simulink model "FrequencyConverter"  (R2025b)
settings: Solver=FixedStepAuto  StartTime=0.0  StopTime=100.0  FixedStep=Ts  RelTol=1e-3
values from neighbouring files (symbols this model uses):
  M_AD_nom = 3500.0    (= 3500)    [constants.m]
  M_max_factor = 2.2    [constants.m]
  poles = 2    [constants.m]
  s_max = 0.05    [constants.m]
settings Model: TunableVars=J_AD,J_ICE,M_AD_nom,P_ballast_nom,P_oil_max,P_oil_min,T_AD_max,T_amb,T_ballast_max,T_cool_max,a_const,ad_fun_acceleration,b_const,k_heat,k_loss,k_loss0,k_rad_AD,k_rad_ballast,k_radiator,omega_ICE_max_prir,omega_ICE_max_run,tau,tau_AD_base,tau_ballast,tau_cool  TunableVarsStorageClass=Auto,Auto,Auto,Auto,Auto,Auto,Auto,Auto,Auto,Auto,Auto,Auto,Auto,Auto,Auto,Auto,Auto,Auto,Auto,Auto,Auto,Auto,Auto,Auto,Auto  TunableVarsTypeQualifier=,,,,,,,,,,,,,,,,,,,,,,,,  Creator=user  LastModifiedBy=user
settings OptimizationCC: DefaultParameterBehavior=Inlined  UseDivisionForNetSlopeComputation=on  GainParamInheritBuiltInType=on  UseFloatMulNetSlope=on  StrengthReduction=on  PassReuseOutputArgsAs=Individual arguments  NoFixptDivByZeroProtection=on  EfficientFloat2IntCast=on  OptimizeBlockOrder=speed  OptimizationPriority=Speed  OptimizationCustomize=off  MultiThreadedLoops=on  AutoScheduleForLoops=on  EfficientTunableParamExpr=on
settings DebuggingCC: ParameterTunabilityLossMsg=error
settings HardwareCC: ProdBitPerLong=64.0  ProdLongLongMode=on  ProdHWDeviceType=Intel->x86-64 (Linux 64)
settings SFSimCC: MATLABDynamicMemAlloc=off  SimTargetLang=C++  SimDLTargetLibrary=mkl-dnn
settings RTWCC: SystemTargetFile=ert.tlc  GenCodeOnly=on  TemplateMakefile=ert_default_tmf  GenerateReport=on  BuildConfiguration=Faster Runs  LaunchReport=on  TargetLang=C++  Description=Embedded Coder
settings CodeAppCC: ForceParamTrailComments=on  IgnoreCustomStorageClasses=off  OperatorAnnotations=on  SimulinkDataObjDesc=on  SFDataObjDesc=on  CustomSymbolStrGlobalVar=rt$N$M  CustomSymbolStrType=$N$M  CustomSymbolStrFcn=$N$M$F  CustomSymbolStrMacro=$N$M  InsertBlockDesc=on
settings ERTTargetCC: InlinedParameterPlacement=Hierarchical  RootIOFormat=Structure reference  ERTCustomFileTemplate=example_file_process.tlc  TargetLangStandard=C++17 (ISO)  GenerateSampleERTMain=on  CodeInterfacePackaging=Reusable function  SupportContinuousTime=on

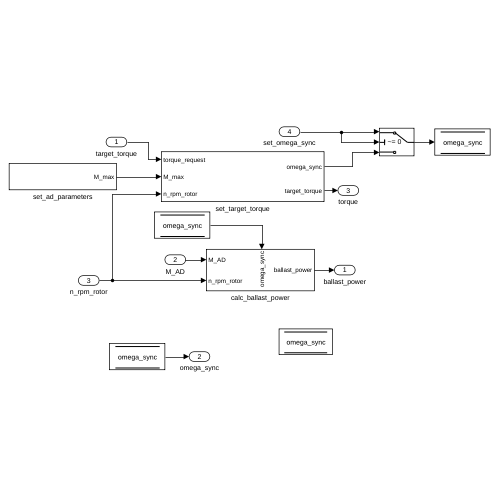
[thumbnail: Simulink's stored preview of the top-level diagram]
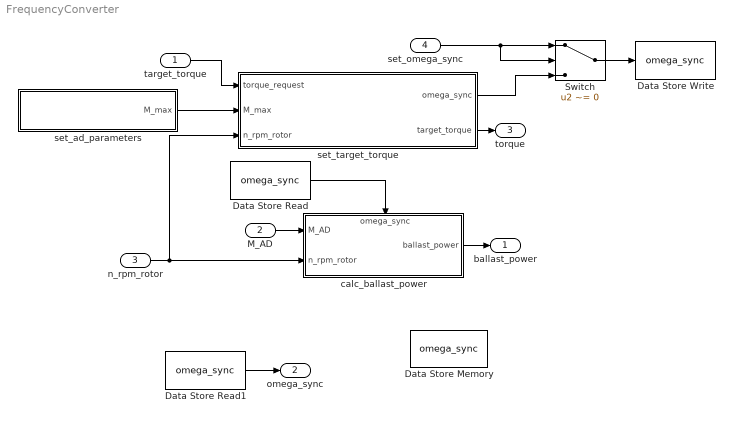
== system FrequencyConverter ==
  target_torque : Inport
  M_AD : Inport  Port=2
  n_rpm_rotor : Inport  Port=3
  set_omega_sync : Inport  Port=4
  Data Store Memory : DataStoreMemory  DataStoreName=omega_sync  WriteAfterWriteMsg=warning  ShowAdditionalParam=off
  Data Store Read : DataStoreRead  DataStoreName=omega_sync  IndexOptions=Index vector (dialog)  Indices=1  OutputSizes=1
  Data Store Read1 : DataStoreRead  DataStoreName=omega_sync  IndexOptions=Index vector (dialog)  Indices=1  OutputSizes=1
  Data Store Write : DataStoreWrite  DataStoreName=omega_sync  IndexOptions=Index vector (dialog)  Indices=1  OutputSizes=1
  Switch : Switch  Criteria=u2 ~= 0  SaturateOnIntegerOverflow=off  InputSameDT=off
  calc_ballast_power : Subsystem
      settings: PortSchema="{\"entries\":[{\"content\":{\"sides\":[{\"content\":{\"connectorIds\":[\"In1\",\"In2\"]},\"type\":\"ConnectorPlacement.EquallySpacedRectSide\",\"uuid\":\"9c23e3e7-388c-4891-afdd-4d1624b884f1\"},{\"content\":{\"connectorIds\":[\"Out1\"],\"side\":\"RIGHT\"},\"type\":\"ConnectorPlacement.EquallySpacedRectSide\",\"uuid\":\"c0260273-0b08-4e98-9658-3297e997359d\"},{\"content\":{\"connectorIds\":[\"In3\"],\"side\":\"TOP\"},\"type\":\"ConnectorPlacement.EquallySpacedRectSide\",\"uuid\":\"b122e6e2-13b5-4687-be80-e20d337b8a3a\"}]},\"type\":\"ConnectorPlacement.EquallySpacedConnector\",\"uuid\":\"625c4f0e-8d47-4f32-9019-3adc0e8607fd\"}],\"packageUris\":[\"http://schema.mathworks.com/mf0/Connector/R2020b\"],\"version\":\"1.0\"}"
  set_ad_parameters : Subsystem
  set_target_torque : Subsystem
  ballast_power : Outport
  omega_sync : Outport  Port=2
  torque : Outport  Port=3
  wires:
  M_AD/1 -> calc_ballast_power/1(M_AD)
  n_rpm_rotor/1 -> set_target_torque/3(n_rpm_rotor), calc_ballast_power/2(n_rpm_rotor)
  calc_ballast_power/1(ballast_power) -> ballast_power/1
  set_ad_parameters/1(M_max) -> set_target_torque/2(M_max)
  target_torque/1 -> set_target_torque/1(torque_request)
  Data Store Read/1 -> calc_ballast_power/3(omega_sync)
  Data Store Read1/1 -> omega_sync/1
  set_target_torque/1(omega_sync) -> Switch/3
  set_omega_sync/1 -> Switch/2, Switch/1
  Switch/1 -> Data Store Write/1
  set_target_torque/2(target_torque) -> torque/1

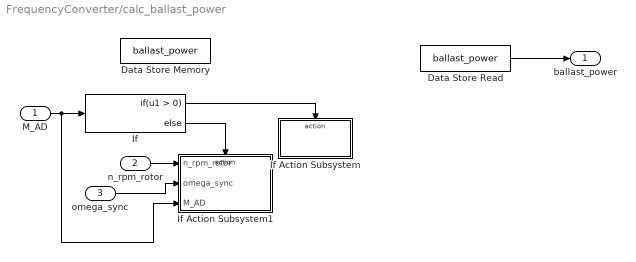
== system FrequencyConverter/calc_ballast_power ==
  M_AD : Inport
  n_rpm_rotor : Inport  Port=2
  omega_sync : Inport  Port=3
  Data Store Memory : DataStoreMemory  DataStoreName=ballast_power  WriteAfterWriteMsg=warning  ShowAdditionalParam=off
  Data Store Read : DataStoreRead  DataStoreName=ballast_power  IndexOptions=Index vector (dialog)  Indices=1  OutputSizes=1
  If : If
  If Action Subsystem : Subsystem  TreatAsAtomicUnit=on
  If Action Subsystem1 : Subsystem  TreatAsAtomicUnit=on
  ballast_power : Outport
  wires:
  Data Store Read/1 -> ballast_power/1
  M_AD/1 -> If Action Subsystem1/3(M_AD), If/1
  If/1 -> If Action Subsystem/Action
  If/2 -> If Action Subsystem1/Action
  n_rpm_rotor/1 -> If Action Subsystem1/1(n_rpm_rotor)
  omega_sync/1 -> If Action Subsystem1/2(omega_sync)

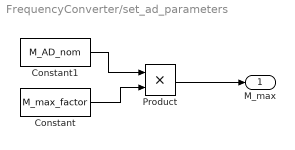
== system FrequencyConverter/set_ad_parameters ==
  Constant : Constant  Value=M_max_factor
  Constant1 : Constant  Value=M_AD_nom
  Product : Product
  M_max : Outport
  wires:
  Constant/1 -> Product/2
  Constant1/1 -> Product/1
  Product/1 -> M_max/1

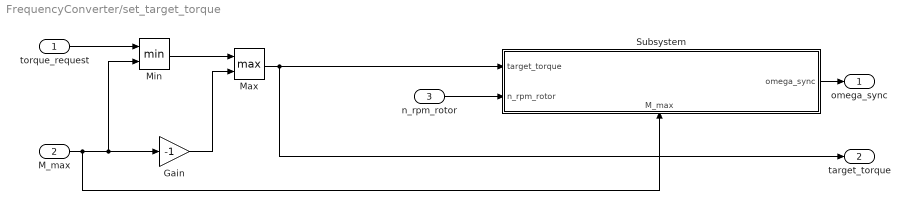
== system FrequencyConverter/set_target_torque ==
  torque_request : Inport
  M_max : Inport  Port=2
  n_rpm_rotor : Inport  Port=3
  Gain : Gain  Gain=-1
  Max : MinMax  Function=max  Inputs=2
  Min : MinMax  Inputs=2
  Subsystem : Subsystem
      settings: PortSchema="{\"entries\":[{\"content\":{\"sides\":[{\"content\":{\"connectorIds\":[\"In1\",\"In2\"]},\"type\":\"ConnectorPlacement.EquallySpacedRectSide\",\"uuid\":\"f5037b0f-1ffd-4c9a-b1c3-4b725bea221f\"},{\"content\":{\"connectorIds\":[\"Out1\"],\"side\":\"RIGHT\"},\"type\":\"ConnectorPlacement.EquallySpacedRectSide\",\"uuid\":\"2266316a-45d6-4ff2-af39-82d45dce8729\"},{\"content\":{\"side\":\"TOP\"},\"type\":\"ConnectorPlacement.EquallySpacedRectSide\",\"uuid\":\"46200062-e85d-4adb-b79b-d00d6ab0e852\"},{\"content\":{\"connectorIds\":[\"In3\"],\"side\":\"BOTTOM\"},\"type\":\"ConnectorPlacement.EquallySpacedRectSide\",\"uuid\":\"97407893-4fba-4239-999b-cdb868f8b31f\"}]},\"type\":\"ConnectorPlacement.EquallySpacedConnector\",\"uuid\":\"87dda9e4-bbd4-43d9-bcb0-f10d68c020c2\"}],\"packageUris\":[\"http://schema.mathworks.com/mf0/Connector/R2020b\"],\"version\":\"1.0\"}"
  omega_sync : Outport
  target_torque : Outport  Port=2
  wires:
  torque_request/1 -> Min/1
  M_max/1 -> Subsystem/3(M_max), Min/2, Gain/1
  Gain/1 -> Max/2
  Max/1 -> target_torque/1, Subsystem/1(target_torque)
  Min/1 -> Max/1
  Subsystem/1(omega_sync) -> omega_sync/1
  n_rpm_rotor/1 -> Subsystem/2(n_rpm_rotor)

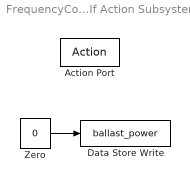
== system FrequencyConverter/calc_ballast_power/If Action Subsystem ==
  Action Port : ActionPort  ActionPortLabel=if(u1 > 0)
  Data Store Write : DataStoreWrite  DataStoreName=ballast_power  IndexOptions=Index vector (dialog)  Indices=1  OutputSizes=1
  Zero : Constant  Value=0  OutDataTypeStr=Inherit: Inherit via back propagation
  wires:
  Zero/1 -> Data Store Write/1

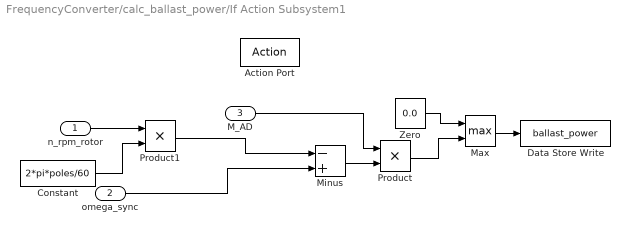
== system FrequencyConverter/calc_ballast_power/If Action Subsystem1 ==
  n_rpm_rotor : Inport
  omega_sync : Inport  Port=2
  M_AD : Inport  Port=3
  Action Port : ActionPort  ActionPortLabel=else
  Constant : Constant  Value=2*pi*poles/60
  Data Store Write : DataStoreWrite  DataStoreName=ballast_power  IndexOptions=Index vector (dialog)  Indices=1  OutputSizes=1
  Max : MinMax  Function=max  Inputs=2
  Minus : Sum  Inputs=-+
  Product : Product
  Product1 : Product
  Zero : Constant  Value=0.0  OutDataTypeStr=Inherit: Inherit via back propagation
  wires:
  Product/1 -> Max/2
  Zero/1 -> Max/1
  Minus/1 -> Product/2
  omega_sync/1 -> Minus/2
  M_AD/1 -> Product/1
  n_rpm_rotor/1 -> Product1/1
  Product1/1 -> Minus/1
  Constant/1 -> Product1/2
  Max/1 -> Data Store Write/1

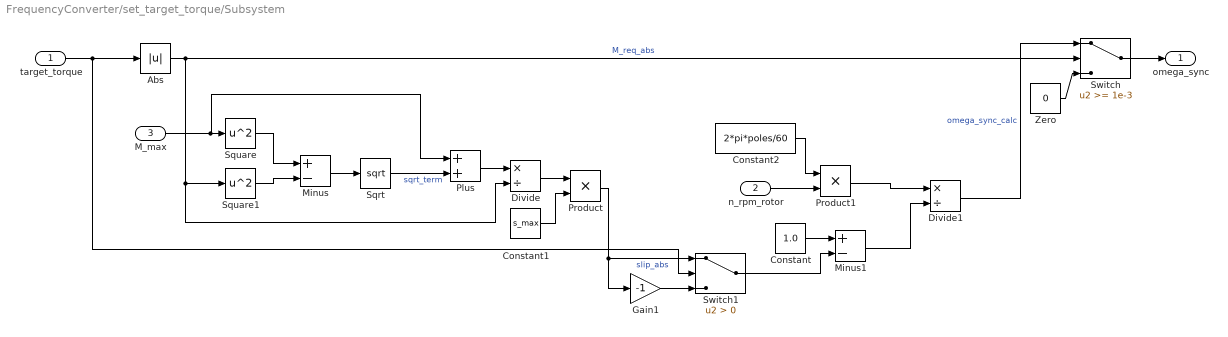
== system FrequencyConverter/set_target_torque/Subsystem ==
  target_torque : Inport
  n_rpm_rotor : Inport  Port=2
  M_max : Inport  Port=3
  Abs : Abs  SaturateOnIntegerOverflow=off
  Constant : Constant  Value=1.0
  Constant1 : Constant  Value=s_max
  Constant2 : Constant  Value=2*pi*poles/60
  Divide : Product  Inputs=*/
  Divide1 : Product  Inputs=*/
  Gain1 : Gain  Gain=-1
  Minus : Sum  Inputs=+-
  Minus1 : Sum  Inputs=+-
  Plus : Sum
  Product : Product
  Product1 : Product
  Sqrt : Sqrt
  Square : Math  Operator=square
  Square1 : Math  Operator=square
  Switch : Switch  Threshold=1e-3  SaturateOnIntegerOverflow=off  InputSameDT=off
  Switch1 : Switch  Criteria=u2 > Threshold  SaturateOnIntegerOverflow=off  InputSameDT=off
  Zero : Constant  Value=0  OutDataTypeStr=Inherit: Inherit via back propagation
  omega_sync : Outport
  wires:
  Switch/1 -> omega_sync/1
  Zero/1 -> Switch/3
  Switch1/1 -> Minus1/2
  M_max/1 -> Plus/1, Square/1
  Constant/1 -> Minus1/1
  Divide1/1 -> Switch/1  "omega_sync_calc"
  Divide/1 -> Product/1
  Sqrt/1 -> Plus/2  "sqrt_term"
  Constant1/1 -> Product/2
  Product/1 -> Switch1/1, Gain1/1  "slip_abs"
  Minus/1 -> Sqrt/1
  Gain1/1 -> Switch1/3
  target_torque/1 -> Switch1/2, Abs/1
  Abs/1 -> Divide/2, Square1/1, Switch/2  "M_req_abs"
  n_rpm_rotor/1 -> Product1/2
  Product1/1 -> Divide1/1
  Plus/1 -> Divide/1
  Square/1 -> Minus/1
  Minus1/1 -> Divide1/2
  Square1/1 -> Minus/2
  Constant2/1 -> Product1/1
